simulink model "FInal_Liu_simulation"  (R2023b)
settings: Solver=ode5  StartTime=0.0  StopTime=2  FixedStep=0.0001  RelTol=1e-3
(part 1 of 2)
settings Model: Creator=amaiani  LastModifiedBy=amaiani

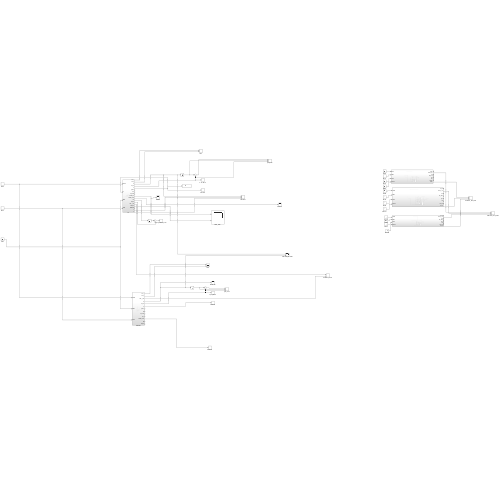
[thumbnail: Simulink's stored preview of the top-level diagram]
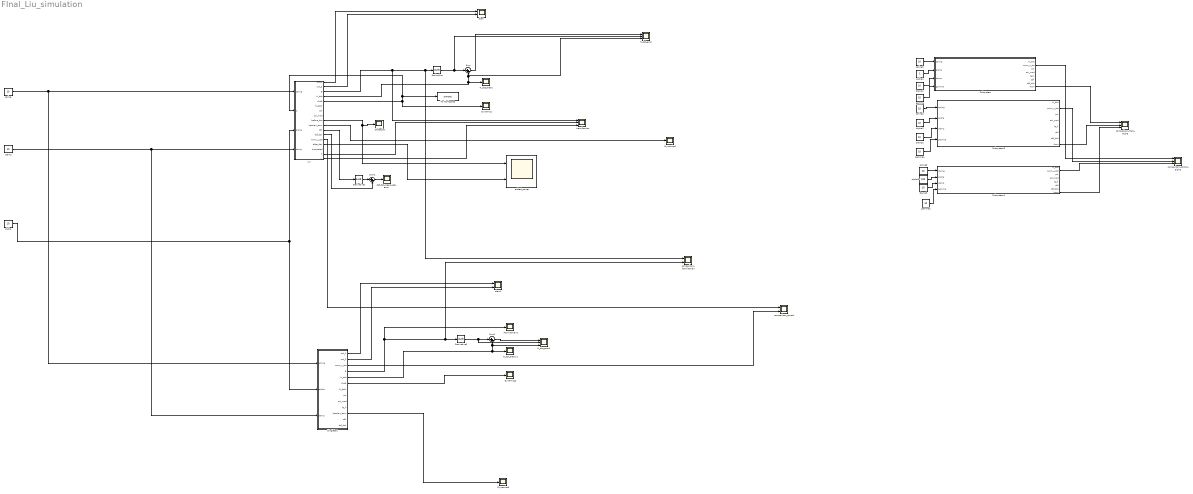
== system FInal_Liu_simulation ==
  Damp{,1..3} (4 alike) : Constant  Value=10
  Derivative : Derivative
  Derivative1 : Derivative
  Derivative2 : Derivative
  Dynamics{,1..3} (4 alike) : Scope
  H_dot_error : Scope  NumInputPorts=3
  H_dot_error1 : Scope  NumInputPorts=3
  H_dot_theory : Scope
  H_dot_theory1 : Scope
  Hamiltonian : Scope  NumInputPorts=3
  Hamiltonian1 : Scope
  Liu : Subsystem
  Singletary : Subsystem
  Subsystem : Subsystem
  Subsystem3 : Subsystem
  Subsystem4 : Subsystem
  Sum : Sum  Inputs=|+-
  Sum1 : Sum  Inputs=|+-
  Sum2 : Sum  Inputs=|+-
  To Workspace : ToWorkspace  VariableName=simout  SampleTime=-1
  added_power : Scope  NumInputPorts=2
  alpha : Constant  Value=10
  alpha1 : Constant
  alpha2 : Constant  Value=10
  alpha3 : Constant  Value=100
  cbf_dot_measured_error : Scope
  comparison_Ham_alpha : Scope  NumInputPorts=3
  comparison_control : Scope  NumInputPorts=2
  comparison_control_alpha : Scope  NumInputPorts=3
  comparison_hamiltonian : Scope  NumInputPorts=2
  dhdqqdot : Scope
  gamma : Constant  Value=10
  gamma1 : Constant  Value=10
  gamma2 : Constant  Value=10
  skew : Scope  NumInputPorts=2
  skew1 : Scope  NumInputPorts=2
  spring{,1..3} (4 alike) : Constant  Value=10
  wires:
  Derivative/1 -> H_dot_error/2, Sum/1
  Sum/1 -> H_dot_error/1
  spring/1 -> Liu/1(spring), Singletary/1(spring)
  Derivative2/1 -> H_dot_error1/2, Sum1/1
  Damp/1 -> Liu/4(damp), Singletary/3(damp)
  Sum1/1 -> H_dot_error1/1
  alpha/1 -> Singletary/2(alpha), Liu/3(alpha)
  Singletary/5(H_dot) -> H_dot_theory1/1, H_dot_error1/3, Sum1/2
  Singletary/4(E) -> Derivative2/1, comparison_hamiltonian/2, Hamiltonian1/1
  Singletary/1(out_1) -> skew1/1
  Singletary/2(out_2) -> skew1/2
  Singletary/3(norm_u_tot) -> comparison_control/2
  Singletary/6(Out6) -> Dynamics2/1
  Singletary/11(hessian_term) -> Dynamics3/1
  Liu/4(H_dot) -> H_dot_theory/1, H_dot_error/3, Sum/2
  Liu/5(Out5) -> Dynamics/1, Liu/2(q), To Workspace/1
  Liu/3(E) -> Derivative/1, comparison_hamiltonian/1, Hamiltonian/1
  Liu/1(out_1) -> skew/1
  Liu/2(out_2) -> skew/2
  Liu/10(hessian_term) -> Dynamics1/1
  Liu/13(norm_u_tot) -> comparison_control/1
  spring1/1 -> Subsystem/1(spring)
  alpha1/1 -> Subsystem/2(alpha)
  Damp1/1 -> Subsystem/3(damp)
  alpha2/1 -> Subsystem3/2(alpha)
  Damp2/1 -> Subsystem3/3(damp)
  spring2/1 -> Subsystem3/1(spring)
  Damp3/1 -> Subsystem4/3(damp)
  alpha3/1 -> Subsystem4/2(alpha)
  spring3/1 -> Subsystem4/1(spring)
  Subsystem/8(Ham) -> comparison_Ham_alpha/1
  Subsystem3/8(Ham) -> comparison_Ham_alpha/2
  Subsystem4/8(Ham) -> comparison_Ham_alpha/3
  Subsystem4/2(norm_u_tot) -> comparison_control_alpha/3
  Subsystem3/2(norm_u_tot) -> comparison_control_alpha/2
  Subsystem/2(norm_u_tot) -> comparison_control_alpha/1
  gamma/1 -> Subsystem/4(gamma)
  gamma1/1 -> Subsystem3/4(gamma)
  gamma2/1 -> Subsystem4/4(gamma)
  Liu/9(before_dot) -> added_power/1, dhdqqdot/1
  Liu/11(cbf) -> Derivative1/1
  Derivative1/1 -> Sum2/1
  Sum2/1 -> cbf_dot_measured_error/1
  Liu/12(cbf_dot) -> Sum2/2
  Liu/14(after_dot) -> added_power/2
  Liu/16(T) -> Hamiltonian/2
  Liu/17(V) -> Hamiltonian/3

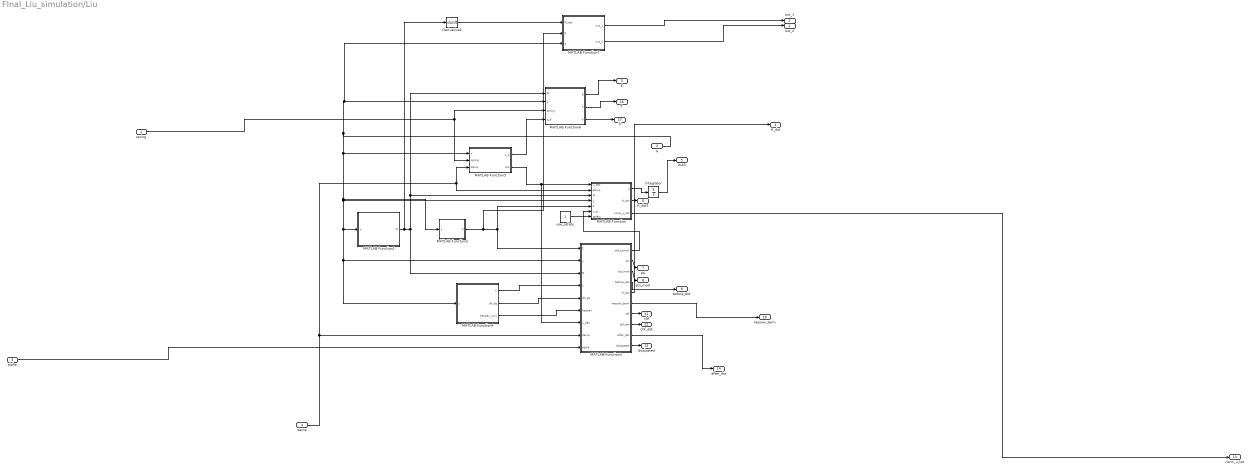
== system FInal_Liu_simulation/Liu ==
  spring : Inport
  q : Inport  Port=2
  alpha : Inport  Port=3
  damp : Inport  Port=4
  Derivative1 : Derivative
  Integrator : Integrator  InitialCondition=[0;0;0;0;0;0]
  MATLAB Function : MATLAB Function  TreatAsAtomicUnit=on
  MATLAB Function1 : MATLAB Function  StartFcn=|  TreatAsAtomicUnit=on
      | % Define numerical values for the parameters
      | xc = 2.5;
      | yc = 2;
      | r = 1;
      | gamma = 2;
      | alpha = 20;
      | 
      | 
      | m1 = 1;
      | m2 = 1;
      | m3 = 1;
      | 
      | 
      | l1 = 1;
      | l2 = 1;
      | l3 = 1;
  MATLAB Function2 : MATLAB Function  StartFcn=|  TreatAsAtomicUnit=on
      | % Define numerical values for the parameters
      | xc = 2.5;
      | yc = 2;
      | r = 1;
      | gamma = 2;
      | alpha = 20;
      | 
      | 
      | m1 = 1;
      | m2 = 1;
      | m3 = 1;
      | 
      | 
      | l1 = 1;
      | l2 = 1;
      | l3 = 1;
  MATLAB Function3 : MATLAB Function  TreatAsAtomicUnit=on
  MATLAB Function4 : MATLAB Function  TreatAsAtomicUnit=on
  MATLAB Function5 : MATLAB Function  TreatAsAtomicUnit=on
  MATLAB Function6 : MATLAB Function  TreatAsAtomicUnit=on
  MATLAB Function7 : MATLAB Function  StartFcn=|  TreatAsAtomicUnit=on
      | % Define numerical values for the parameters
      | xc = 2.5;
      | yc = 2;
      | r = 1;
      | gamma = 2;
      | alpha = 20;
      | 
      | 
      | m1 = 1;
      | m2 = 1;
      | m3 = 1;
      | 
      | 
      | l1 = 1;
      | l2 = 1;
      | l3 = 1;
  use_safety : Constant
  out_1 : Outport
  out_2 : Outport  Port=2
  E : Outport  Port=3
  H_dot : Outport  Port=4
  Out5 : Outport  Port=5
  H_dot1 : Outport  Port=6
  psi : Outport  Port=7
  psi_mod : Outport  Port=8
  before_dot : Outport  Port=9
  hessian_term : Outport  Port=10
  cbf : Outport  Port=11
  cbf_dot : Outport  Port=12
  norm_u_tot : Outport  Port=13
  after_dot : Outport  Port=14
  dissipated : Outport  Port=15
  T : Outport  Port=16
  V : Outport  Port=17
  wires:
  MATLAB Function3/8(cbf_dot) -> cbf_dot/1
  MATLAB Function3/2(psi) -> psi/1
  MATLAB Function3/7(cbf) -> cbf/1
  MATLAB Function/3(norm_u_tot) -> norm_u_tot/1
  MATLAB Function/2(H_dot) -> H_dot1/1
  Integrator/1 -> Out5/1
  MATLAB Function4/3(hessian_sym) -> MATLAB Function3/6(hessian)
  MATLAB Function1/1(M) -> Derivative1/1, MATLAB Function6/1(M), MATLAB Function/3(M), MATLAB Function3/3(M)
  MATLAB Function4/2(dh_dq) -> MATLAB Function3/5(dh_dq)
  MATLAB Function7/1(out_1) -> out_1/1
  alpha/1 -> MATLAB Function3/9(alpha)
  MATLAB Function6/1(E) -> E/1
  MATLAB Function3/3(psi_mod) -> psi_mod/1
  MATLAB Function7/2(out_2) -> out_2/1
  use_safety/1 -> MATLAB Function/7(safety)
  MATLAB Function3/4(before_dot) -> before_dot/1
  Derivative1/1 -> MATLAB Function7/1(M_dot)
  MATLAB Function5/1(q_d) -> MATLAB Function6/4(q_d)
  MATLAB Function3/5(H_dot) -> H_dot/1
  MATLAB Function/1(y) -> Integrator/1
  MATLAB Function3/1(cbf_control) -> MATLAB Function/6(u_sc)
  MATLAB Function2/1(C) -> MATLAB Function/5(C), MATLAB Function3/1(C), MATLAB Function7/2(S)
  MATLAB Function4/1(h) -> MATLAB Function3/4(h)
  spring/1 -> MATLAB Function6/3(spring), MATLAB Function5/2(spring)
  MATLAB Function5/2(out) -> MATLAB Function3/7(u_des), MATLAB Function/1(u_des)
  MATLAB Function3/6(hessian_term) -> hessian_term/1
  q/1 -> MATLAB Function7/3(q), MATLAB Function6/2(y), MATLAB Function5/1(y), MATLAB Function2/1(y), MATLAB Function4/1(y), MATLAB Function3/2(y), MATLAB Function1/1(y), MATLAB Function/4("y ")
  damp/1 -> MATLAB Function/2(damp), MATLAB Function5/3(damp), MATLAB Function3/8(damp)
  MATLAB Function3/9(after_dot) -> after_dot/1
  MATLAB Function3/10(dissipated) -> dissipated/1
  MATLAB Function6/2(T) -> T/1
  MATLAB Function6/3(V) -> V/1

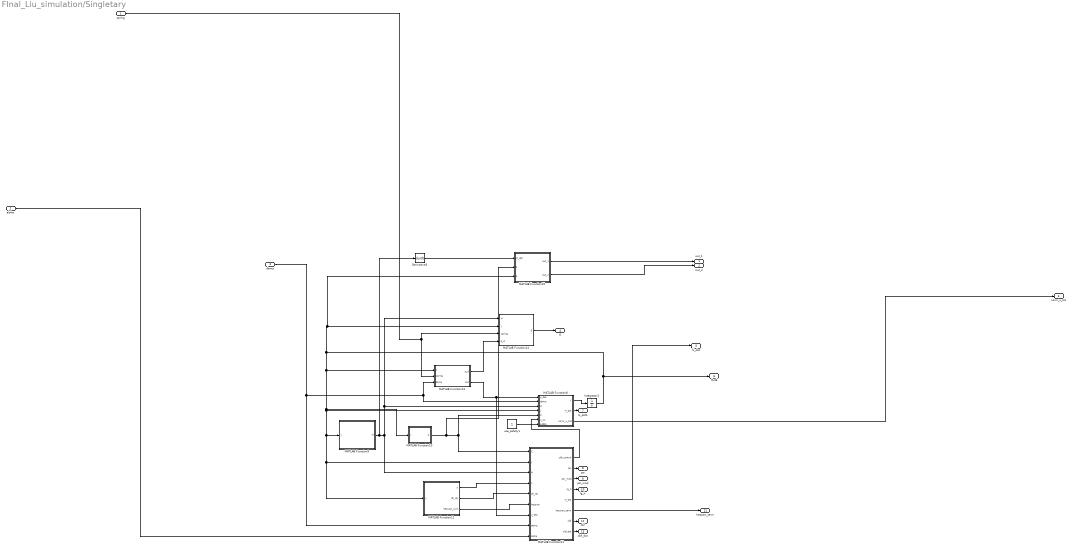
== system FInal_Liu_simulation/Singletary ==
  spring : Inport
  alpha : Inport  Port=2
  damp : Inport  Port=3
  Derivative3 : Derivative
  Integrator1 : Integrator  InitialCondition=[0;0;0;0;0;0]
  MATLAB Function10 : MATLAB Function  StartFcn=|  TreatAsAtomicUnit=on
      | % Define numerical values for the parameters
      | xc = 2.5;
      | yc = 2;
      | r = 1;
      | gamma = 2;
      | alpha = 20;
      | 
      | 
      | m1 = 1;
      | m2 = 1;
      | m3 = 1;
      | 
      | 
      | l1 = 1;
      | l2 = 1;
      | l3 = 1;
  MATLAB Function11 : MATLAB Function  TreatAsAtomicUnit=on
  MATLAB Function12 : MATLAB Function  TreatAsAtomicUnit=on
  MATLAB Function13 : MATLAB Function  TreatAsAtomicUnit=on
  MATLAB Function14 : MATLAB Function  TreatAsAtomicUnit=on
  MATLAB Function15 : MATLAB Function  StartFcn=|  TreatAsAtomicUnit=on
      | % Define numerical values for the parameters
      | xc = 2.5;
      | yc = 2;
      | r = 1;
      | gamma = 2;
      | alpha = 20;
      | 
      | 
      | m1 = 1;
      | m2 = 1;
      | m3 = 1;
      | 
      | 
      | l1 = 1;
      | l2 = 1;
      | l3 = 1;
  MATLAB Function8 : MATLAB Function  TreatAsAtomicUnit=on
  MATLAB Function9 : MATLAB Function  StartFcn=|  TreatAsAtomicUnit=on
      | % Define numerical values for the parameters
      | xc = 2.5;
      | yc = 2;
      | r = 1;
      | gamma = 2;
      | alpha = 20;
      | 
      | 
      | m1 = 1;
      | m2 = 1;
      | m3 = 1;
      | 
      | 
      | l1 = 1;
      | l2 = 1;
      | l3 = 1;
  use_safety1 : Constant
  out_1 : Outport
  out_2 : Outport  Port=2
  norm_u_tot : Outport  Port=3
  E : Outport  Port=4
  H_dot : Outport  Port=5
  Out6 : Outport  Port=6
  H_dot1 : Outport  Port=7
  psi : Outport  Port=8
  psi_mod : Outport  Port=9
  lg_h : Outport  Port=10
  hessian_term : Outport  Port=11
  cbf : Outport  Port=12
  cbf_dot : Outport  Port=13
  wires:
  MATLAB Function11/2(psi) -> psi/1
  MATLAB Function11/4(lg_h) -> lg_h/1
  MATLAB Function11/7(cbf) -> cbf/1
  MATLAB Function8/2(H_dot) -> H_dot1/1
  MATLAB Function11/5(H_dot) -> H_dot/1
  MATLAB Function11/6(hessian_term) -> hessian_term/1
  MATLAB Function14/1(E) -> E/1
  MATLAB Function8/3(norm_u_tot) -> norm_u_tot/1
  MATLAB Function12/3(hessian_sym) -> MATLAB Function11/6(hessian)
  Derivative3/1 -> MATLAB Function15/1(M_dot)
  MATLAB Function12/1(h) -> MATLAB Function11/4(h)
  MATLAB Function8/1(y) -> Integrator1/1
  MATLAB Function11/3(psi_mod) -> psi_mod/1
  alpha/1 -> MATLAB Function11/9(alpha)
  spring/1 -> MATLAB Function13/2(spring), MATLAB Function14/3(spring)
  MATLAB Function10/1(C) -> MATLAB Function8/5(C), MATLAB Function11/1(C), MATLAB Function15/2(S)
  MATLAB Function13/1(q_d) -> MATLAB Function14/4(q_d)
  MATLAB Function11/1(cbf_control) -> MATLAB Function8/6(u_sc)
  MATLAB Function15/2(out_2) -> out_2/1
  Integrator1/1 -> Out6/1, MATLAB Function15/3(q), MATLAB Function14/2(y), MATLAB Function13/1(y), MATLAB Function10/1(y), MATLAB Function12/1(y), MATLAB Function11/2(y), MATLAB Function9/1(y), MATLAB Function8/4("y ")
  MATLAB Function15/1(out_1) -> out_1/1
  damp/1 -> MATLAB Function11/8(damp), MATLAB Function8/2(damp), MATLAB Function13/3(damp)
  MATLAB Function12/2(dh_dq) -> MATLAB Function11/5(dh_dq)
  MATLAB Function13/2(out) -> MATLAB Function11/7(u_des), MATLAB Function8/1(u_des)
  MATLAB Function11/8(cbf_dot) -> cbf_dot/1
  use_safety1/1 -> MATLAB Function8/7(safety)
  MATLAB Function9/1(M) -> Derivative3/1, MATLAB Function14/1(M), MATLAB Function8/3(M), MATLAB Function11/3(M)

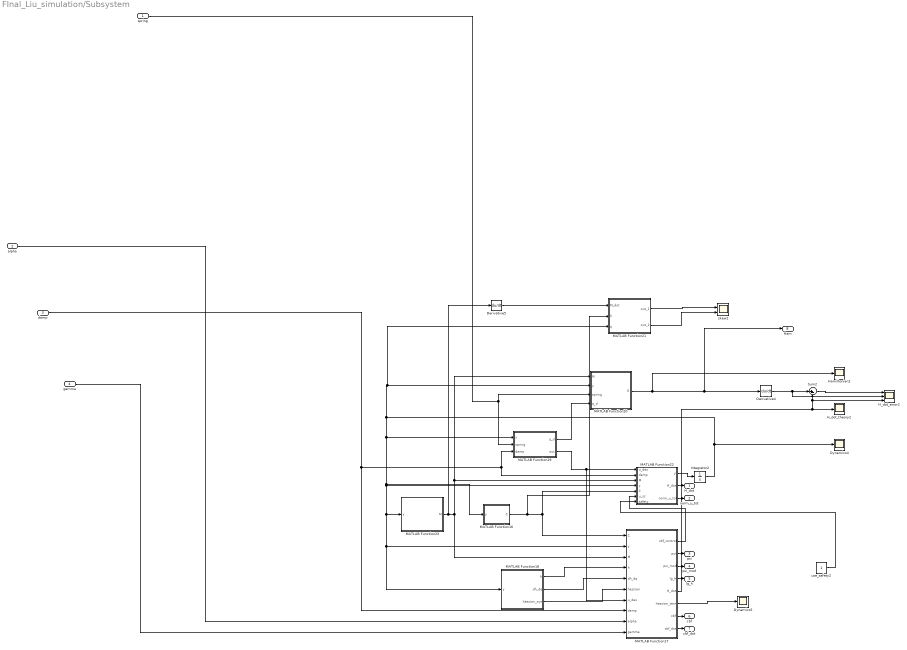
== system FInal_Liu_simulation/Subsystem ==
  spring : Inport
  alpha : Inport  Port=2
  damp : Inport  Port=3
  gamma : Inport  Port=4
  Derivative4 : Derivative
  Derivative5 : Derivative
  Dynamics4 : Scope
  Dynamics5 : Scope
  H_dot_error2 : Scope  NumInputPorts=3
  H_dot_theory2 : Scope
  Hamiltonian2 : Scope
  Integrator2 : Integrator  InitialCondition=[0;0;0;0;0;0]
  MATLAB Function16 : MATLAB Function  StartFcn=|  TreatAsAtomicUnit=on
      | % Define numerical values for the parameters
      | xc = 2.5;
      | yc = 2;
      | r = 1;
      | gamma = 2;
      | alpha = 20;
      | 
      | 
      | m1 = 1;
      | m2 = 1;
      | m3 = 1;
      | 
      | 
      | l1 = 1;
      | l2 = 1;
      | l3 = 1;
  MATLAB Function17 : MATLAB Function  TreatAsAtomicUnit=on
  MATLAB Function18 : MATLAB Function  TreatAsAtomicUnit=on
  MATLAB Function19 : MATLAB Function  TreatAsAtomicUnit=on
  MATLAB Function20 : MATLAB Function  TreatAsAtomicUnit=on
  MATLAB Function21 : MATLAB Function  StartFcn=|  TreatAsAtomicUnit=on
      | % Define numerical values for the parameters
      | xc = 2.5;
      | yc = 2;
      | r = 1;
      | gamma = 2;
      | alpha = 20;
      | 
      | 
      | m1 = 1;
      | m2 = 1;
      | m3 = 1;
      | 
      | 
      | l1 = 1;
      | l2 = 1;
      | l3 = 1;
  MATLAB Function22 : MATLAB Function  TreatAsAtomicUnit=on
  MATLAB Function23 : MATLAB Function  StartFcn=|  TreatAsAtomicUnit=on
      | % Define numerical values for the parameters
      | xc = 2.5;
      | yc = 2;
      | r = 1;
      | gamma = 2;
      | alpha = 20;
      | 
      | 
      | m1 = 1;
      | m2 = 1;
      | m3 = 1;
      | 
      | 
      | l1 = 1;
      | l2 = 1;
      | l3 = 1;
  Sum2 : Sum  Inputs=|+-
  skew2 : Scope  NumInputPorts=2
  use_safety2 : Constant
  H_dot : Outport
  norm_u_tot : Outport  Port=2
  psi : Outport  Port=3
  psi_mod : Outport  Port=4
  lg_h : Outport  Port=5
  cbf : Outport  Port=6
  cbf_dot : Outport  Port=7
  Ham : Outport  Port=8
  wires:
  MATLAB Function17/3(psi_mod) -> psi_mod/1
  MATLAB Function17/8(cbf_dot) -> cbf_dot/1
  MATLAB Function17/4(lg_h) -> lg_h/1
  alpha/1 -> MATLAB Function17/9(alpha)
  MATLAB Function17/2(psi) -> psi/1
  MATLAB Function17/1(cbf_control) -> MATLAB Function22/6(u_sc)
  MATLAB Function23/1(M) -> Derivative5/1, MATLAB Function20/1(M), MATLAB Function22/3(M), MATLAB Function17/3(M)
  use_safety2/1 -> MATLAB Function22/7(safety)
  MATLAB Function22/1(y) -> Integrator2/1
  MATLAB Function17/7(cbf) -> cbf/1
  Sum2/1 -> H_dot_error2/1
  Derivative4/1 -> H_dot_error2/2, Sum2/1
  MATLAB Function22/3(norm_u_tot) -> norm_u_tot/1
  MATLAB Function18/2(dh_dq) -> MATLAB Function17/5(dh_dq)
  Derivative5/1 -> MATLAB Function21/1(M_dot)
  MATLAB Function19/2(out) -> MATLAB Function17/7(u_des), MATLAB Function22/1(u_des)
  MATLAB Function17/6(hessian_term) -> Dynamics5/1
  MATLAB Function18/3(hessian_sym) -> MATLAB Function17/6(hessian)
  MATLAB Function21/1(out_1) -> skew2/1
  MATLAB Function21/2(out_2) -> skew2/2
  MATLAB Function19/1(q_d) -> MATLAB Function20/4(q_d)
  MATLAB Function22/2(H_dot) -> H_dot/1
  damp/1 -> MATLAB Function17/8(damp), MATLAB Function22/2(damp), MATLAB Function19/3(damp)
  MATLAB Function20/1(E) -> Ham/1, Derivative4/1, Hamiltonian2/1
  Integrator2/1 -> Dynamics4/1, MATLAB Function21/3(q), MATLAB Function20/2(y), MATLAB Function19/1(y), MATLAB Function16/1(y), MATLAB Function18/1(y), MATLAB Function17/2(y), MATLAB Function23/1(y), MATLAB Function22/4("y ")
  MATLAB Function18/1(h) -> MATLAB Function17/4(h)
  spring/1 -> MATLAB Function19/2(spring), MATLAB Function20/3(spring)
  MATLAB Function16/1(C) -> MATLAB Function22/5(C), MATLAB Function17/1(C), MATLAB Function21/2(S)
  MATLAB Function17/5(H_dot) -> H_dot_theory2/1, H_dot_error2/3, Sum2/2
  gamma/1 -> MATLAB Function17/10(gamma)

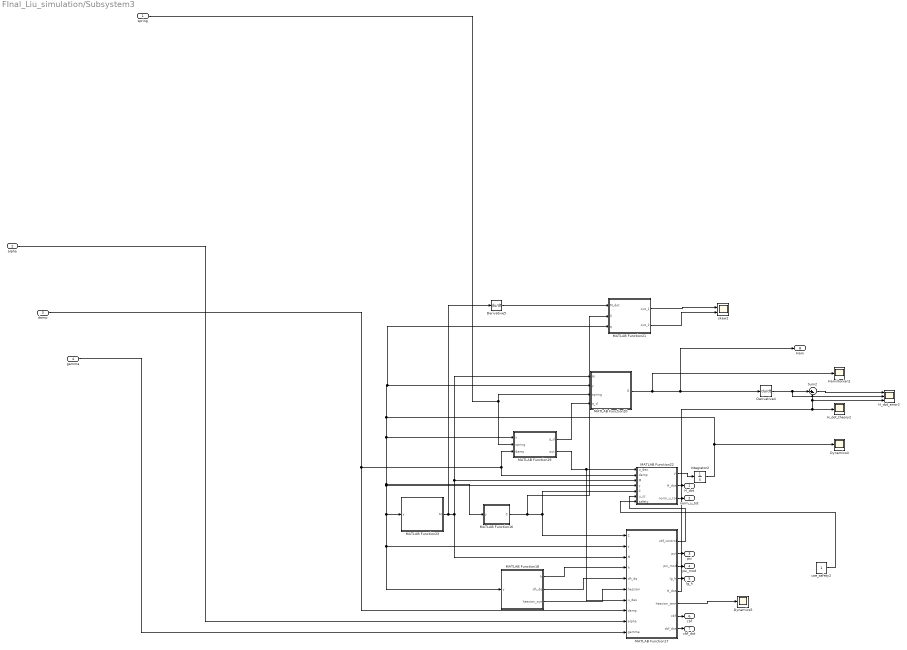
== system FInal_Liu_simulation/Subsystem3 ==
  spring : Inport
  alpha : Inport  Port=2
  damp : Inport  Port=3
  gamma : Inport  Port=4
  Derivative4 : Derivative
  Derivative5 : Derivative
  Dynamics4 : Scope
  Dynamics5 : Scope
  H_dot_error2 : Scope  NumInputPorts=3
  H_dot_theory2 : Scope
  Hamiltonian2 : Scope
  Integrator2 : Integrator  InitialCondition=[0;0;0;0;0;0]
  MATLAB Function16 : MATLAB Function  StartFcn=|  TreatAsAtomicUnit=on
      | % Define numerical values for the parameters
      | xc = 2.5;
      | yc = 2;
      | r = 1;
      | gamma = 2;
      | alpha = 20;
      | 
      | 
      | m1 = 1;
      | m2 = 1;
      | m3 = 1;
      | 
      | 
      | l1 = 1;
      | l2 = 1;
      | l3 = 1;
  MATLAB Function17 : MATLAB Function  TreatAsAtomicUnit=on
  MATLAB Function18 : MATLAB Function  TreatAsAtomicUnit=on
  MATLAB Function19 : MATLAB Function  TreatAsAtomicUnit=on
  MATLAB Function20 : MATLAB Function  TreatAsAtomicUnit=on
  MATLAB Function21 : MATLAB Function  StartFcn=|  TreatAsAtomicUnit=on
      | % Define numerical values for the parameters
      | xc = 2.5;
      | yc = 2;
      | r = 1;
      | gamma = 2;
      | alpha = 20;
      | 
      | 
      | m1 = 1;
      | m2 = 1;
      | m3 = 1;
      | 
      | 
      | l1 = 1;
      | l2 = 1;
      | l3 = 1;
  MATLAB Function22 : MATLAB Function  TreatAsAtomicUnit=on
  MATLAB Function23 : MATLAB Function  StartFcn=|  TreatAsAtomicUnit=on
      | % Define numerical values for the parameters
      | xc = 2.5;
      | yc = 2;
      | r = 1;
      | gamma = 2;
      | alpha = 20;
      | 
      | 
      | m1 = 1;
      | m2 = 1;
      | m3 = 1;
      | 
      | 
      | l1 = 1;
      | l2 = 1;
      | l3 = 1;
  Sum2 : Sum  Inputs=|+-
  skew2 : Scope  NumInputPorts=2
  use_safety2 : Constant
  H_dot : Outport
  norm_u_tot : Outport  Port=2
  psi : Outport  Port=3
  psi_mod : Outport  Port=4
  lg_h : Outport  Port=5
  cbf : Outport  Port=6
  cbf_dot : Outport  Port=7
  Ham : Outport  Port=8
  wires:
  MATLAB Function17/3(psi_mod) -> psi_mod/1
  MATLAB Function17/8(cbf_dot) -> cbf_dot/1
  MATLAB Function17/4(lg_h) -> lg_h/1
  alpha/1 -> MATLAB Function17/9(alpha)
  MATLAB Function17/2(psi) -> psi/1
  MATLAB Function17/1(cbf_control) -> MATLAB Function22/6(u_sc)
  MATLAB Function23/1(M) -> Derivative5/1, MATLAB Function20/1(M), MATLAB Function22/3(M), MATLAB Function17/3(M)
  use_safety2/1 -> MATLAB Function22/7(safety)
  MATLAB Function22/1(y) -> Integrator2/1
  MATLAB Function17/7(cbf) -> cbf/1
  Sum2/1 -> H_dot_error2/1
  Derivative4/1 -> H_dot_error2/2, Sum2/1
  MATLAB Function22/3(norm_u_tot) -> norm_u_tot/1
  MATLAB Function18/2(dh_dq) -> MATLAB Function17/5(dh_dq)
  Derivative5/1 -> MATLAB Function21/1(M_dot)
  MATLAB Function19/2(out) -> MATLAB Function17/7(u_des), MATLAB Function22/1(u_des)
  MATLAB Function17/6(hessian_term) -> Dynamics5/1
  MATLAB Function18/3(hessian_sym) -> MATLAB Function17/6(hessian)
  MATLAB Function21/1(out_1) -> skew2/1
  MATLAB Function21/2(out_2) -> skew2/2
  MATLAB Function19/1(q_d) -> MATLAB Function20/4(q_d)
  MATLAB Function22/2(H_dot) -> H_dot/1
  damp/1 -> MATLAB Function17/8(damp), MATLAB Function22/2(damp), MATLAB Function19/3(damp)
  MATLAB Function20/1(E) -> Ham/1, Derivative4/1, Hamiltonian2/1
  Integrator2/1 -> Dynamics4/1, MATLAB Function21/3(q), MATLAB Function20/2(y), MATLAB Function19/1(y), MATLAB Function16/1(y), MATLAB Function18/1(y), MATLAB Function17/2(y), MATLAB Function23/1(y), MATLAB Function22/4("y ")
  MATLAB Function18/1(h) -> MATLAB Function17/4(h)
  spring/1 -> MATLAB Function19/2(spring), MATLAB Function20/3(spring)
  MATLAB Function16/1(C) -> MATLAB Function22/5(C), MATLAB Function17/1(C), MATLAB Function21/2(S)
  MATLAB Function17/5(H_dot) -> H_dot_theory2/1, H_dot_error2/3, Sum2/2
  gamma/1 -> MATLAB Function17/10(gamma)

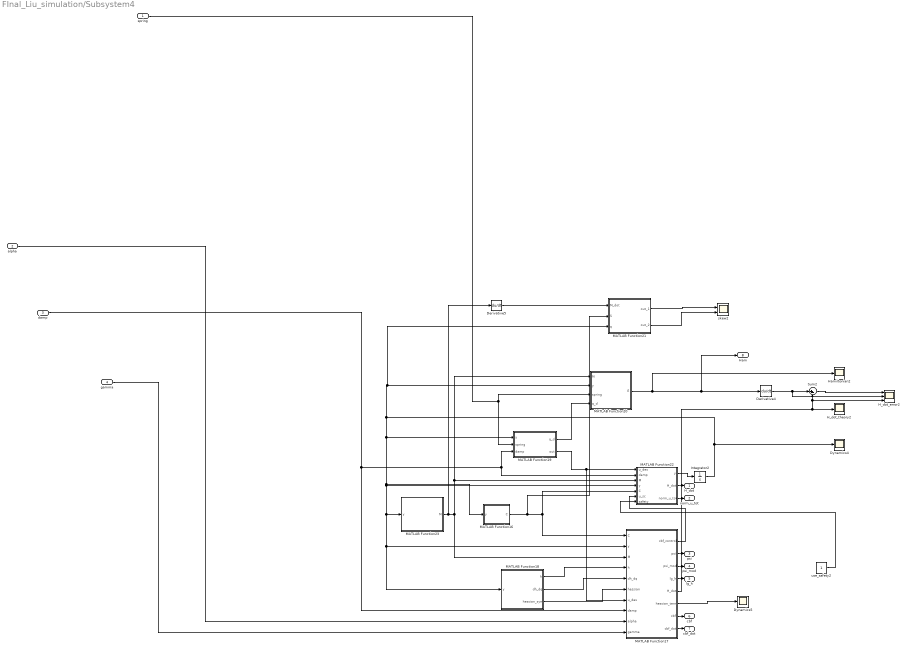
== system FInal_Liu_simulation/Subsystem4 ==
  spring : Inport
  alpha : Inport  Port=2
  damp : Inport  Port=3
  gamma : Inport  Port=4
  Derivative4 : Derivative
  Derivative5 : Derivative
  Dynamics4 : Scope
  Dynamics5 : Scope
  H_dot_error2 : Scope  NumInputPorts=3
  H_dot_theory2 : Scope
  Hamiltonian2 : Scope
  Integrator2 : Integrator  InitialCondition=[0;0;0;0;0;0]
  MATLAB Function16 : MATLAB Function  StartFcn=|  TreatAsAtomicUnit=on
      | % Define numerical values for the parameters
      | xc = 2.5;
      | yc = 2;
      | r = 1;
      | gamma = 2;
      | alpha = 20;
      | 
      | 
      | m1 = 1;
      | m2 = 1;
      | m3 = 1;
      | 
      | 
      | l1 = 1;
      | l2 = 1;
      | l3 = 1;
  MATLAB Function17 : MATLAB Function  TreatAsAtomicUnit=on
  MATLAB Function18 : MATLAB Function  TreatAsAtomicUnit=on
  MATLAB Function19 : MATLAB Function  TreatAsAtomicUnit=on
  MATLAB Function20 : MATLAB Function  TreatAsAtomicUnit=on
  MATLAB Function21 : MATLAB Function  StartFcn=|  TreatAsAtomicUnit=on
      | % Define numerical values for the parameters
      | xc = 2.5;
      | yc = 2;
      | r = 1;
      | gamma = 2;
      | alpha = 20;
      | 
      | 
      | m1 = 1;
      | m2 = 1;
      | m3 = 1;
      | 
      | 
      | l1 = 1;
      | l2 = 1;
      | l3 = 1;
  MATLAB Function22 : MATLAB Function  TreatAsAtomicUnit=on
  MATLAB Function23 : MATLAB Function  StartFcn=|  TreatAsAtomicUnit=on
      | % Define numerical values for the parameters
      | xc = 2.5;
      | yc = 2;
      | r = 1;
      | gamma = 2;
      | alpha = 20;
      | 
      | 
      | m1 = 1;
      | m2 = 1;
      | m3 = 1;
      | 
      | 
      | l1 = 1;
      | l2 = 1;
      | l3 = 1;
  Sum2 : Sum  Inputs=|+-
  skew2 : Scope  NumInputPorts=2
  use_safety2 : Constant
  H_dot : Outport
  norm_u_tot : Outport  Port=2
  psi : Outport  Port=3
  psi_mod : Outport  Port=4
  lg_h : Outport  Port=5
  cbf : Outport  Port=6
  cbf_dot : Outport  Port=7
  Ham : Outport  Port=8
  wires:
  MATLAB Function17/3(psi_mod) -> psi_mod/1
  MATLAB Function17/8(cbf_dot) -> cbf_dot/1
  MATLAB Function17/4(lg_h) -> lg_h/1
  alpha/1 -> MATLAB Function17/9(alpha)
  MATLAB Function17/2(psi) -> psi/1
  MATLAB Function17/1(cbf_control) -> MATLAB Function22/6(u_sc)
  MATLAB Function23/1(M) -> Derivative5/1, MATLAB Function20/1(M), MATLAB Function22/3(M), MATLAB Function17/3(M)
  use_safety2/1 -> MATLAB Function22/7(safety)
  MATLAB Function22/1(y) -> Integrator2/1
  MATLAB Function17/7(cbf) -> cbf/1
  Sum2/1 -> H_dot_error2/1
  Derivative4/1 -> H_dot_error2/2, Sum2/1
  MATLAB Function22/3(norm_u_tot) -> norm_u_tot/1
  MATLAB Function18/2(dh_dq) -> MATLAB Function17/5(dh_dq)
  Derivative5/1 -> MATLAB Function21/1(M_dot)
  MATLAB Function19/2(out) -> MATLAB Function17/7(u_des), MATLAB Function22/1(u_des)
  MATLAB Function17/6(hessian_term) -> Dynamics5/1
  MATLAB Function18/3(hessian_sym) -> MATLAB Function17/6(hessian)
  MATLAB Function21/1(out_1) -> skew2/1
  MATLAB Function21/2(out_2) -> skew2/2
  MATLAB Function19/1(q_d) -> MATLAB Function20/4(q_d)
  MATLAB Function22/2(H_dot) -> H_dot/1
  damp/1 -> MATLAB Function17/8(damp), MATLAB Function22/2(damp), MATLAB Function19/3(damp)
  MATLAB Function20/1(E) -> Ham/1, Derivative4/1, Hamiltonian2/1
  Integrator2/1 -> Dynamics4/1, MATLAB Function21/3(q), MATLAB Function20/2(y), MATLAB Function19/1(y), MATLAB Function16/1(y), MATLAB Function18/1(y), MATLAB Function17/2(y), MATLAB Function23/1(y), MATLAB Function22/4("y ")
  MATLAB Function18/1(h) -> MATLAB Function17/4(h)
  spring/1 -> MATLAB Function19/2(spring), MATLAB Function20/3(spring)
  MATLAB Function16/1(C) -> MATLAB Function22/5(C), MATLAB Function17/1(C), MATLAB Function21/2(S)
  MATLAB Function17/5(H_dot) -> H_dot_theory2/1, H_dot_error2/3, Sum2/2
  gamma/1 -> MATLAB Function17/10(gamma)

== matlab function FInal_Liu_simulation/Liu/MATLAB Function6 ==
  data: M input; E output; y input; spring input; q_d input; T output; V output
function [E,T,V] = energy(M,y,spring, q_d)
    q = y(1:3);
    dq = y(4:6);
    
    T = 0.5 * (dq' * M * dq) ;
    V =0.5 * spring *(q-q_d)' * (q-q_d);
    E = T + V;

== matlab function FInal_Liu_simulation/Liu/MATLAB Function7 ==
  data: M_dot input; out_1 output; S input; q input; out_2 output


function [out_1, out_2] = M_dot_coriolis_check(M_dot,S, q)
    dq = reshape(q(4:6),[3,1]);
    
    q1 = q(1);
    q2 = q(2);
    q3 = q(3);
    dq1 = q(4);
    dq2 = q(5);
    dq3 = q(6);

    check = M_dot - 2 * S;


    out_1 = dq' * check * dq;


    M_dot_formula =   [        - dq2*(sin(q2 + q3) + 3*sin(q2)) - dq3*(sin(q2 + q3) + sin(q3)), - dq3*(sin(q2 + q3)/2 + sin(q3)) - dq2*(sin(q2 + q3)/2 + (3*sin(q2))/2), - (dq2*sin(q2 + q3))/2 - dq3*(sin(q2 + q3)/2 + sin(q3)/2);
- dq3*(sin(q2 + q3)/2 + sin(q3)) - dq2*(sin(q2 + q3)/2 + (3*sin(q2))/2),                                                            -dq3*sin(q3),                                          -(dq3*sin(q3))/2;
              - (dq2*sin(q2 + q3))/2 - dq3*(sin(q2 + q3)/2 + sin(q3)/2),                                                        -(dq3*sin(q3))/2,                                                         0];
 

    
    out_2 = dq' * (M_dot_formula - 2 * S) * dq;
end

== matlab function FInal_Liu_simulation/Singletary/MATLAB Function10 ==
  data: y input; C output
function C = coriolis(y)

    q1 = y(1);
    q2 = y(2);
    q3 = y(3);
    dq1 = y(4);
    dq2 = y(5);
    dq3 = y(6);


    C = [- dq2*(sin(q2 + q3)/2 + (3*sin(q2))/2) - dq3*(sin(q2 + q3)/2 + sin(q3)/2), - dq1*(sin(q2 + q3)/2 + (3*sin(q2))/2) - dq2*(sin(q2 + q3)/2 + (3*sin(q2))/2) - dq3*(sin(q2 + q3)/2 + sin(q3)/2), - dq1*(sin(q2 + q3)/2 + sin(q3)/2) - dq2*(sin(q2 + q3)/2 + sin(q3)/2) - dq3*(sin(q2 + q3)/2 + sin(q3)/2);
                dq1*(sin(q2 + q3)/2 + (3*sin(q2))/2) - (dq3*sin(q3))/2,                                                                                                 -(dq3*sin(q3))/2,                                                    - (dq1*sin(q3))/2 - (dq2*sin(q3))/2 - (dq3*sin(q3))/2;
                       dq1*(sin(q2 + q3)/2 + sin(q3)/2) + (dq2*sin(q3))/2,                                                                                (dq1*sin(q3))/2 + (dq2*sin(q3))/2,                                                                                                        0];

== matlab function FInal_Liu_simulation/Singletary/MATLAB Function11 ==
  data: C input; y input; cbf_control output; M input; h input; dh_dq input; hessian input; u_des input; psi output; psi_mod output; lg_h output; H_dot output; damp input; hessian_term output; cbf output; cbf_dot output; alpha input

function [cbf_control, psi, psi_mod,lg_h, H_dot, hessian_term, cbf, cbf_dot]= CBF(C, y, M, h, dh_dq, hessian, u_des, damp, alpha)
% Define numerical values for the parameters
    xc = 2.5;
    yc = 2;
    r = 1;
    gamma = 2;

    
    m1 = 1;
    m2 = 1;
    m3 = 1;
    
    l1 = 1;
    l2 = 1;
    l3 = 1;
    
    q = reshape(y(1:3),[3,1]);
    dq = reshape(y(4:6),[3,1]);
    dh_dq = reshape(dh_dq,[1,3]);

    LIU = 0;

    if LIU == 1

    
        cbf = alpha * h + dh_dq * dq;
        lg_h = zeros(1,3);
        cbf_dot_prior = alpha .* dh_dq * dq + dq' * hessian * dq + dh_dq * (inv(M)* (-C * dq + u_des));
        psi = cbf_dot_prior + gamma .* cbf;
        if psi<0
            lg_h = dh_dq * inv(M);
            cbf_control =  - lg_h' /(lg_h * lg_h')  .* psi;
            
        else
            cbf_control = zeros(3,1);
        end
        cbf_dot = alpha .* dh_dq * dq + dq' * hessian * dq + dh_dq * inv(M)* (-C * dq + u_des+ cbf_control);
        psi_mod = cbf_dot + gamma .* cbf;

        H_dot = dq' * cbf_control - dq' * damp * dq;

        hessian_term = dq' * hessian * dq;
    
    else
        KE = 0.5 * dq' * M * dq;
        cbf = alpha * h - KE;
        lg_h = zeros(1,3);
        cbf_dot_prior = alpha .* dh_dq * dq - dq' * inv(M) * u_des;
        psi = cbf_dot_prior + gamma .* cbf;
        if psi<0
            lg_h = -dq';
            cbf_control =  dq /(dq'*dq)  .* psi;
        else
            cbf_control = zeros(3,1);
        end
        cbf_dot =  alpha .* dh_dq * dq - dq' * inv(M) * (u_des+cbf_control) ;
        psi_mod = cbf_dot + gamma .* cbf;

        H_dot = dq' * cbf_control - dq' * damp * dq;


        hessian_term = 0;
        
    end
    
end

== matlab function FInal_Liu_simulation/Singletary/MATLAB Function12 ==
  data: y input; h output; dh_dq output; hessian_sym output
function [h, dh_dq, hessian_sym] = obstacle(y)
    % Define numerical values for the parameters
    xc = 2.5;
    yc = 2;
    r = 1;

    l1 = 1;
    l2 = 1;
    l3 = 1;
    
    % Compute the end-effector position using forward kinematics
    q1 = y(1);
    q2 = y(2);
    q3 = y(3);
    
    x_ee = l1 * cos(q1) + l2 * cos(q1 + q2) + l3 * cos(q1 + q2 + q3);
    y_ee = l1 * sin(q1) + l2 * sin(q1 + q2) + l3 * sin(q1 + q2 + q3);
    
    % Compute the control barrier function h
    h = (xc - x_ee)^2 + (yc - y_ee)^2 - r^2;
    
    % Define the expressions for dh_dq and hessian_sym
    dh_dq = [2*(cos(q1 + q2 + q3) + cos(q1 + q2) + cos(q1))*(sin(q1 + q2 + q3) + sin(q1 + q2) + sin(q1) - 2) - 2*(sin(q1 + q2 + q3) + sin(q1 + q2) + sin(q1))*(cos(q1 + q2 + q3) + cos(q1 + q2) + cos(q1) - 5/2), 2*(cos(q1 + q2 + q3) + cos(q1 + q2))*(sin(q1 + q2 + q3) + sin(q1 + q2) + sin(q1) - 2) - 2*(sin(q1 + q2 + q3) + sin(q1 + q2))*(cos(q1 + q2 + q3) + cos(q1 + q2) + cos(q1) - 5/2), 2*cos(q1 + q2 + q3)*(sin(q1 + q2 + q3) + sin(q1 + q2) + sin(q1) - 2) - 2*sin(q1 + q2 + q3)*(cos(q1 + q2 + q3) + cos(q1 + q2) + cos(q1) - 5/2)];


    hessian_sym = [                                              2*(cos(q1 + q2 + q3) + cos(q1 + q2) + cos(q1))^2 - 2*(cos(q1 + q2 + q3) + cos(q1 + q2) + cos(q1))*(cos(q1 + q2 + q3) + cos(q1 + q2) + cos(q1) - 5/2) + 2*(sin(q1 + q2 + q3) + sin(q1 + q2) + sin(q1))^2 - 2*(sin(q1 + q2 + q3) + sin(q1 + q2) + sin(q1))*(sin(q1 + q2 + q3) + sin(q1 + q2) + sin(q1) - 2), 2*(cos(q1 + q2 + q3) + cos(q1 + q2))*(cos(q1 + q2 + q3) + cos(q1 + q2) + cos(q1)) - 2*(cos(q1 + q2 + q3) + cos(q1 + q2))*(cos(q1 + q2 + q3) + cos(q1 + q2) + cos(q1) - 5/2) + 2*(sin(q1 + q2 + q3) + sin(q1 + q2))*(sin(q1 + q2 + q3) + sin(q1 + q2) + sin(q1)) - 2*(sin(q1 + q2 + q3) + sin(q1 + q2))*(sin(q1 + q2 + q3) + sin(q1 + q2) + sin(q1) - 2), 2*cos(q1 + q2 + q3)*(cos(q1 + q2 + q3) + cos(q1 + q2) + cos(q1)) - 2*cos(q1 + q2 + q3)*(cos(q1 + q2 + q3) + cos(q1 + q2) + cos(q1) - 5/2) + 2*sin(q1 + q2 + q3)*(sin(q1 + q2 + q3) + sin(q1 + q2) + sin(q1)) - 2*sin(q1 + q2 + q3)*(sin(q1 + q2 + q3) + sin(q1 + q2) + sin(q1) - 2);
        2*(cos(q1 + q2 + q3) + cos(q1 + q2))*(cos(q1 + q2 + q3) + cos(q1 + q2) + cos(q1)) - 2*(cos(q1 + q2 + q3) + cos(q1 + q2))*(cos(q1 + q2 + q3) + cos(q1 + q2) + cos(q1) - 5/2) + 2*(sin(q1 + q2 + q3) + sin(q1 + q2))*(sin(q1 + q2 + q3) + sin(q1 + q2) + sin(q1)) - 2*(sin(q1 + q2 + q3) + sin(q1 + q2))*(sin(q1 + q2 + q3) + sin(q1 + q2) + sin(q1) - 2),                                                                                       2*(cos(q1 + q2 + q3) + cos(q1 + q2))^2 - 2*(cos(q1 + q2 + q3) + cos(q1 + q2))*(cos(q1 + q2 + q3) + cos(q1 + q2) + cos(q1) - 5/2) + 2*(sin(q1 + q2 + q3) + sin(q1 + q2))^2 - 2*(sin(q1 + q2 + q3) + sin(q1 + q2))*(sin(q1 + q2 + q3) + sin(q1 + q2) + sin(q1) - 2),                     2*cos(q1 + q2 + q3)*(cos(q1 + q2 + q3) + cos(q1 + q2)) - 2*cos(q1 + q2 + q3)*(cos(q1 + q2 + q3) + cos(q1 + q2) + cos(q1) - 5/2) - 2*sin(q1 + q2 + q3)*(sin(q1 + q2 + q3) + sin(q1 + q2) + sin(q1) - 2) + 2*sin(q1 + q2 + q3)*(sin(q1 + q2 + q3) + sin(q1 + q2));
                                                                            2*cos(q1 + q2 + q3)*(cos(q1 + q2 + q3) + cos(q1 + q2) + cos(q1)) - 2*cos(q1 + q2 + q3)*(cos(q1 + q2 + q3) + cos(q1 + q2) + cos(q1) - 5/2) + 2*sin(q1 + q2 + q3)*(sin(q1 + q2 + q3) + sin(q1 + q2) + sin(q1)) - 2*sin(q1 + q2 + q3)*(sin(q1 + q2 + q3) + sin(q1 + q2) + sin(q1) - 2),                                                                                         2*cos(q1 + q2 + q3)*(cos(q1 + q2 + q3) + cos(q1 + q2)) - 2*cos(q1 + q2 + q3)*(cos(q1 + q2 + q3) + cos(q1 + q2) + cos(q1) - 5/2) - 2*sin(q1 + q2 + q3)*(sin(q1 + q2 + q3) + sin(q1 + q2) + sin(q1) - 2) + 2*sin(q1 + q2 + q3)*(sin(q1 + q2 + q3) + sin(q1 + q2)),                                                                                       2*cos(q1 + q2 + q3)^2 - 2*cos(q1 + q2 + q3)*(cos(q1 + q2 + q3) + cos(q1 + q2) + cos(q1) - 5/2) + 2*sin(q1 + q2 + q3)^2 - 2*sin(q1 + q2 + q3)*(sin(q1 + q2 + q3) + sin(q1 + q2) + sin(q1) - 2)];
     

    % d = eig(hessian_sym)
    % isposdef = all(d >= 0);
    % 
    % assert(isposdef, 'error hessian');
end

== matlab function FInal_Liu_simulation/Singletary/MATLAB Function13 ==
  data: q_d output; y input; spring input; out output; damp input
function [q_d, out] = u_des(y, spring, damp)


    q = reshape(y(1:3),[3,1]);
    dq = reshape(y(4:6),[3,1]);

    q_d = [pi; 0; pi/4];
    
    out =  - damp * dq - spring * (q-q_d);

== matlab function FInal_Liu_simulation/Singletary/MATLAB Function14 ==
  data: M input; E output; y input; spring input; q_d input
function E = energy(M,y,spring, q_d)
    q = y(1:3);
    dq = y(4:6);
    

    E = 0.5 * (dq' * M * dq) + 0.5 * spring *(q-q_d)' * (q-q_d);

== matlab function FInal_Liu_simulation/Singletary/MATLAB Function15 ==
  data: M_dot input; out_1 output; S input; q input; out_2 output


function [out_1, out_2] = M_dot_coriolis_check(M_dot,S, q)
    dq = reshape(q(4:6),[3,1]);
    
    q1 = q(1);
    q2 = q(2);
    q3 = q(3);
    dq1 = q(4);
    dq2 = q(5);
    dq3 = q(6);

    check = M_dot - 2 * S;


    out_1 = dq' * check * dq;


    M_dot_formula =   [        - dq2*(sin(q2 + q3) + 3*sin(q2)) - dq3*(sin(q2 + q3) + sin(q3)), - dq3*(sin(q2 + q3)/2 + sin(q3)) - dq2*(sin(q2 + q3)/2 + (3*sin(q2))/2), - (dq2*sin(q2 + q3))/2 - dq3*(sin(q2 + q3)/2 + sin(q3)/2);
- dq3*(sin(q2 + q3)/2 + sin(q3)) - dq2*(sin(q2 + q3)/2 + (3*sin(q2))/2),                                                            -dq3*sin(q3),                                          -(dq3*sin(q3))/2;
              - (dq2*sin(q2 + q3))/2 - dq3*(sin(q2 + q3)/2 + sin(q3)/2),                                                        -(dq3*sin(q3))/2,                                                         0];
 

    
    out_2 = dq' * (M_dot_formula - 2 * S) * dq;
end

== matlab function FInal_Liu_simulation/Singletary/MATLAB Function8 ==
  data: u_des input; damp input; M input; y input; y output; C input; H_dot output; u_sc input; safety input; norm_u_tot output
function [y,H_dot,norm_u_tot]= dynamics(u_des, damp , M,y, C, u_sc, safety)
    
    q = reshape(y(1:3),[3,1]);
    dq = reshape(y(4:6),[3,1]);



    [~, p] = chol(M);
    decision = (p == 0);

    assert(decision, 'Inertia matrix is not positive definite');
    
    u_tot = u_des + safety * u_sc;
    norm_u_tot=norm(u_tot);
    ddq = inv(M) * (u_tot - C * dq ); % + u_sc

    H_dot = - dq' * damp * dq;

    y = [dq; ddq];

== matlab function FInal_Liu_simulation/Singletary/MATLAB Function9 ==
  data: y input; M output
function M = inertia_M(y)

    q1 = y(1);
    q2 = y(2);
    q3 = y(3);

    M  = [        cos(q2 + q3) + 3*cos(q2) + cos(q3) + 4, cos(q2 + q3)/2 + (3*cos(q2))/2 + cos(q3) + 5/3, cos(q2 + q3)/2 + cos(q3)/2 + 1/3;
cos(q2 + q3)/2 + (3*cos(q2))/2 + cos(q3) + 5/3,                                  cos(q3) + 5/3,                  cos(q3)/2 + 1/3;
              cos(q2 + q3)/2 + cos(q3)/2 + 1/3,                                cos(q3)/2 + 1/3,                              1/3];

== matlab function FInal_Liu_simulation/Subsystem/MATLAB Function16 ==
  data: y input; C output
function C = coriolis(y)

    q1 = y(1);
    q2 = y(2);
    q3 = y(3);
    dq1 = y(4);
    dq2 = y(5);
    dq3 = y(6);


    C = [- dq2*(sin(q2 + q3)/2 + (3*sin(q2))/2) - dq3*(sin(q2 + q3)/2 + sin(q3)/2), - dq1*(sin(q2 + q3)/2 + (3*sin(q2))/2) - dq2*(sin(q2 + q3)/2 + (3*sin(q2))/2) - dq3*(sin(q2 + q3)/2 + sin(q3)/2), - dq1*(sin(q2 + q3)/2 + sin(q3)/2) - dq2*(sin(q2 + q3)/2 + sin(q3)/2) - dq3*(sin(q2 + q3)/2 + sin(q3)/2);
                dq1*(sin(q2 + q3)/2 + (3*sin(q2))/2) - (dq3*sin(q3))/2,                                                                                                 -(dq3*sin(q3))/2,                                                    - (dq1*sin(q3))/2 - (dq2*sin(q3))/2 - (dq3*sin(q3))/2;
                       dq1*(sin(q2 + q3)/2 + sin(q3)/2) + (dq2*sin(q3))/2,                                                                                (dq1*sin(q3))/2 + (dq2*sin(q3))/2,                                                                                                        0];

== matlab function FInal_Liu_simulation/Subsystem/MATLAB Function17 ==
  data: C input; y input; cbf_control output; M input; h input; dh_dq input; hessian input; u_des input; psi output; psi_mod output; lg_h output; H_dot output; damp input; hessian_term output; cbf output; cbf_dot output; alpha input; gamma input

function [cbf_control, psi, psi_mod,lg_h, H_dot, hessian_term, cbf, cbf_dot]= CBF(C, y, M, h, dh_dq, hessian, u_des, damp, alpha, gamma)
% Define numerical values for the parameters
    xc = 2.5;
    yc = 2;
    r = 1;

    
    m1 = 1;
    m2 = 1;
    m3 = 1;
    
    l1 = 1;
    l2 = 1;
    l3 = 1;
    
    q = reshape(y(1:3),[3,1]);
    dq = reshape(y(4:6),[3,1]);
    dh_dq = reshape(dh_dq,[1,3]);

    LIU = 1;

    if LIU == 1

    
        cbf = alpha * h + dh_dq * dq;
        lg_h = zeros(1,3);
        cbf_dot_prior = alpha .* dh_dq * dq + dq' * hessian * dq + dh_dq * (inv(M)* (-C * dq + u_des));
        psi = cbf_dot_prior + gamma .* cbf;
        if psi<0
            lg_h = dh_dq * inv(M);
            cbf_control =  - lg_h' /(lg_h * lg_h')  .* psi;
            
        else
            cbf_control = zeros(3,1);
        end
        cbf_dot = alpha .* dh_dq * dq + dq' * hessian * dq + dh_dq * inv(M)* (-C * dq + u_des+ cbf_control);
        psi_mod = cbf_dot + gamma .* cbf;

        H_dot = dq' * cbf_control - dq' * damp * dq;

        hessian_term = dq' * hessian * dq;
    
    else
        KE = 0.5 * dq' * M * dq;
        cbf = alpha * h - KE;
        lg_h = zeros(1,3);
        cbf_dot_prior = alpha .* dh_dq * dq - dq' * inv(M) * u_des;
        psi = cbf_dot_prior + gamma .* cbf;
        if psi<0
            lg_h = -dq';
            cbf_control =  dq /(dq'*dq)  .* psi;
        else
            cbf_control = zeros(3,1);
        end
        cbf_dot =  alpha .* dh_dq * dq - dq' * inv(M) * (u_des+cbf_control) ;
        psi_mod = cbf_dot + gamma .* cbf;

        H_dot = dq' * cbf_control - dq' * damp * dq;


        hessian_term = 0;
        
    end
    
end

== matlab function FInal_Liu_simulation/Subsystem/MATLAB Function18 ==
  data: y input; h output; dh_dq output; hessian_sym output
function [h, dh_dq, hessian_sym] = obstacle(y)
    % Define numerical values for the parameters
    xc = 2.5;
    yc = 2;
    r = 1;

    l1 = 1;
    l2 = 1;
    l3 = 1;
    
    % Compute the end-effector position using forward kinematics
    q1 = y(1);
    q2 = y(2);
    q3 = y(3);
    
    x_ee = l1 * cos(q1) + l2 * cos(q1 + q2) + l3 * cos(q1 + q2 + q3);
    y_ee = l1 * sin(q1) + l2 * sin(q1 + q2) + l3 * sin(q1 + q2 + q3);
    
    % Compute the control barrier function h
    h = (xc - x_ee)^2 + (yc - y_ee)^2 - r^2;
    
    % Define the expressions for dh_dq and hessian_sym
    dh_dq = [2*(cos(q1 + q2 + q3) + cos(q1 + q2) + cos(q1))*(sin(q1 + q2 + q3) + sin(q1 + q2) + sin(q1) - 2) - 2*(sin(q1 + q2 + q3) + sin(q1 + q2) + sin(q1))*(cos(q1 + q2 + q3) + cos(q1 + q2) + cos(q1) - 5/2), 2*(cos(q1 + q2 + q3) + cos(q1 + q2))*(sin(q1 + q2 + q3) + sin(q1 + q2) + sin(q1) - 2) - 2*(sin(q1 + q2 + q3) + sin(q1 + q2))*(cos(q1 + q2 + q3) + cos(q1 + q2) + cos(q1) - 5/2), 2*cos(q1 + q2 + q3)*(sin(q1 + q2 + q3) + sin(q1 + q2) + sin(q1) - 2) - 2*sin(q1 + q2 + q3)*(cos(q1 + q2 + q3) + cos(q1 + q2) + cos(q1) - 5/2)];


    hessian_sym = [                                              2*(cos(q1 + q2 + q3) + cos(q1 + q2) + cos(q1))^2 - 2*(cos(q1 + q2 + q3) + cos(q1 + q2) + cos(q1))*(cos(q1 + q2 + q3) + cos(q1 + q2) + cos(q1) - 5/2) + 2*(sin(q1 + q2 + q3) + sin(q1 + q2) + sin(q1))^2 - 2*(sin(q1 + q2 + q3) + sin(q1 + q2) + sin(q1))*(sin(q1 + q2 + q3) + sin(q1 + q2) + sin(q1) - 2), 2*(cos(q1 + q2 + q3) + cos(q1 + q2))*(cos(q1 + q2 + q3) + cos(q1 + q2) + cos(q1)) - 2*(cos(q1 + q2 + q3) + cos(q1 + q2))*(cos(q1 + q2 + q3) + cos(q1 + q2) + cos(q1) - 5/2) + 2*(sin(q1 + q2 + q3) + sin(q1 + q2))*(sin(q1 + q2 + q3) + sin(q1 + q2) + sin(q1)) - 2*(sin(q1 + q2 + q3) + sin(q1 + q2))*(sin(q1 + q2 + q3) + sin(q1 + q2) + sin(q1) - 2), 2*cos(q1 + q2 + q3)*(cos(q1 + q2 + q3) + cos(q1 + q2) + cos(q1)) - 2*cos(q1 + q2 + q3)*(cos(q1 + q2 + q3) + cos(q1 + q2) + cos(q1) - 5/2) + 2*sin(q1 + q2 + q3)*(sin(q1 + q2 + q3) + sin(q1 + q2) + sin(q1)) - 2*sin(q1 + q2 + q3)*(sin(q1 + q2 + q3) + sin(q1 + q2) + sin(q1) - 2);
        2*(cos(q1 + q2 + q3) + cos(q1 + q2))*(cos(q1 + q2 + q3) + cos(q1 + q2) + cos(q1)) - 2*(cos(q1 + q2 + q3) + cos(q1 + q2))*(cos(q1 + q2 + q3) + cos(q1 + q2) + cos(q1) - 5/2) + 2*(sin(q1 + q2 + q3) + sin(q1 + q2))*(sin(q1 + q2 + q3) + sin(q1 + q2) + sin(q1)) - 2*(sin(q1 + q2 + q3) + sin(q1 + q2))*(sin(q1 + q2 + q3) + sin(q1 + q2) + sin(q1) - 2),                                                                                       2*(cos(q1 + q2 + q3) + cos(q1 + q2))^2 - 2*(cos(q1 + q2 + q3) + cos(q1 + q2))*(cos(q1 + q2 + q3) + cos(q1 + q2) + cos(q1) - 5/2) + 2*(sin(q1 + q2 + q3) + sin(q1 + q2))^2 - 2*(sin(q1 + q2 + q3) + sin(q1 + q2))*(sin(q1 + q2 + q3) + sin(q1 + q2) + sin(q1) - 2),                     2*cos(q1 + q2 + q3)*(cos(q1 + q2 + q3) + cos(q1 + q2)) - 2*cos(q1 + q2 + q3)*(cos(q1 + q2 + q3) + cos(q1 + q2) + cos(q1) - 5/2) - 2*sin(q1 + q2 + q3)*(sin(q1 + q2 + q3) + sin(q1 + q2) + sin(q1) - 2) + 2*sin(q1 + q2 + q3)*(sin(q1 + q2 + q3) + sin(q1 + q2));
                                                                            2*cos(q1 + q2 + q3)*(cos(q1 + q2 + q3) + cos(q1 + q2) + cos(q1)) - 2*cos(q1 + q2 + q3)*(cos(q1 + q2 + q3) + cos(q1 + q2) + cos(q1) - 5/2) + 2*sin(q1 + q2 + q3)*(sin(q1 + q2 + q3) + sin(q1 + q2) + sin(q1)) - 2*sin(q1 + q2 + q3)*(sin(q1 + q2 + q3) + sin(q1 + q2) + sin(q1) - 2),                                                                                         2*cos(q1 + q2 + q3)*(cos(q1 + q2 + q3) + cos(q1 + q2)) - 2*cos(q1 + q2 + q3)*(cos(q1 + q2 + q3) + cos(q1 + q2) + cos(q1) - 5/2) - 2*sin(q1 + q2 + q3)*(sin(q1 + q2 + q3) + sin(q1 + q2) + sin(q1) - 2) + 2*sin(q1 + q2 + q3)*(sin(q1 + q2 + q3) + sin(q1 + q2)),                                                                                       2*cos(q1 + q2 + q3)^2 - 2*cos(q1 + q2 + q3)*(cos(q1 + q2 + q3) + cos(q1 + q2) + cos(q1) - 5/2) + 2*sin(q1 + q2 + q3)^2 - 2*sin(q1 + q2 + q3)*(sin(q1 + q2 + q3) + sin(q1 + q2) + sin(q1) - 2)];
     

    % d = eig(hessian_sym)
    % isposdef = all(d >= 0);
    % 
    % assert(isposdef, 'error hessian');
end

== matlab function FInal_Liu_simulation/Subsystem/MATLAB Function19 ==
  data: q_d output; y input; spring input; out output; damp input
function [q_d, out] = u_des(y, spring, damp)


    q = reshape(y(1:3),[3,1]);
    dq = reshape(y(4:6),[3,1]);

    q_d = [pi; 0; pi/4];
    
    out =  - damp * dq - spring * (q-q_d);

== matlab function FInal_Liu_simulation/Subsystem/MATLAB Function20 ==
  data: M input; E output; y input; spring input; q_d input
function E = energy(M,y,spring, q_d)
    q = y(1:3);
    dq = y(4:6);
    

    E = 0.5 * (dq' * M * dq) + 0.5 * spring *(q-q_d)' * (q-q_d);

== matlab function FInal_Liu_simulation/Subsystem/MATLAB Function21 ==
  data: M_dot input; out_1 output; S input; q input; out_2 output


function [out_1, out_2] = M_dot_coriolis_check(M_dot,S, q)
    dq = reshape(q(4:6),[3,1]);
    
    q1 = q(1);
    q2 = q(2);
    q3 = q(3);
    dq1 = q(4);
    dq2 = q(5);
    dq3 = q(6);

    check = M_dot - 2 * S;


    out_1 = dq' * check * dq;


    M_dot_formula =   [        - dq2*(sin(q2 + q3) + 3*sin(q2)) - dq3*(sin(q2 + q3) + sin(q3)), - dq3*(sin(q2 + q3)/2 + sin(q3)) - dq2*(sin(q2 + q3)/2 + (3*sin(q2))/2), - (dq2*sin(q2 + q3))/2 - dq3*(sin(q2 + q3)/2 + sin(q3)/2);
- dq3*(sin(q2 + q3)/2 + sin(q3)) - dq2*(sin(q2 + q3)/2 + (3*sin(q2))/2),                                                            -dq3*sin(q3),                                          -(dq3*sin(q3))/2;
              - (dq2*sin(q2 + q3))/2 - dq3*(sin(q2 + q3)/2 + sin(q3)/2),                                                        -(dq3*sin(q3))/2,                                                         0];
 

    
    out_2 = dq' * (M_dot_formula - 2 * S) * dq;
end

== matlab function FInal_Liu_simulation/Liu/MATLAB Function1 ==
  data: y input; M output
function M = inertia_M(y)

    q1 = y(1);
    q2 = y(2);
    q3 = y(3);

    M  = [        cos(q2 + q3) + 3*cos(q2) + cos(q3) + 4, cos(q2 + q3)/2 + (3*cos(q2))/2 + cos(q3) + 5/3, cos(q2 + q3)/2 + cos(q3)/2 + 1/3;
cos(q2 + q3)/2 + (3*cos(q2))/2 + cos(q3) + 5/3,                                  cos(q3) + 5/3,                  cos(q3)/2 + 1/3;
              cos(q2 + q3)/2 + cos(q3)/2 + 1/3,                                cos(q3)/2 + 1/3,                              1/3];

    assert(isequal(M, M'),'error')

== matlab function FInal_Liu_simulation/Subsystem/MATLAB Function22 ==
  data: u_des input; damp input; M input; y input; y output; C input; H_dot output; u_sc input; safety input; norm_u_tot output
function [y,H_dot,norm_u_tot]= dynamics(u_des, damp , M,y, C, u_sc, safety)
    
    q = reshape(y(1:3),[3,1]);
    dq = reshape(y(4:6),[3,1]);



    [~, p] = chol(M);
    decision = (p == 0);

    assert(decision, 'Inertia matrix is not positive definite');
    
    u_tot = u_des + safety * u_sc;
    norm_u_tot=norm(u_tot);
    ddq = inv(M) * (u_tot - C * dq ); % + u_sc

    H_dot = - dq' * damp * dq;

    y = [dq; ddq];

== matlab function FInal_Liu_simulation/Subsystem/MATLAB Function23 ==
  data: y input; M output
function M = inertia_M(y)

    q1 = y(1);
    q2 = y(2);
    q3 = y(3);

    M  = [        cos(q2 + q3) + 3*cos(q2) + cos(q3) + 4, cos(q2 + q3)/2 + (3*cos(q2))/2 + cos(q3) + 5/3, cos(q2 + q3)/2 + cos(q3)/2 + 1/3;
cos(q2 + q3)/2 + (3*cos(q2))/2 + cos(q3) + 5/3,                                  cos(q3) + 5/3,                  cos(q3)/2 + 1/3;
              cos(q2 + q3)/2 + cos(q3)/2 + 1/3,                                cos(q3)/2 + 1/3,                              1/3];

== matlab function FInal_Liu_simulation/Subsystem3/MATLAB Function16 ==
  data: y input; C output
function C = coriolis(y)

    q1 = y(1);
    q2 = y(2);
    q3 = y(3);
    dq1 = y(4);
    dq2 = y(5);
    dq3 = y(6);


    C = [- dq2*(sin(q2 + q3)/2 + (3*sin(q2))/2) - dq3*(sin(q2 + q3)/2 + sin(q3)/2), - dq1*(sin(q2 + q3)/2 + (3*sin(q2))/2) - dq2*(sin(q2 + q3)/2 + (3*sin(q2))/2) - dq3*(sin(q2 + q3)/2 + sin(q3)/2), - dq1*(sin(q2 + q3)/2 + sin(q3)/2) - dq2*(sin(q2 + q3)/2 + sin(q3)/2) - dq3*(sin(q2 + q3)/2 + sin(q3)/2);
                dq1*(sin(q2 + q3)/2 + (3*sin(q2))/2) - (dq3*sin(q3))/2,                                                                                                 -(dq3*sin(q3))/2,                                                    - (dq1*sin(q3))/2 - (dq2*sin(q3))/2 - (dq3*sin(q3))/2;
                       dq1*(sin(q2 + q3)/2 + sin(q3)/2) + (dq2*sin(q3))/2,                                                                                (dq1*sin(q3))/2 + (dq2*sin(q3))/2,                                                                                                        0];

== matlab function FInal_Liu_simulation/Subsystem3/MATLAB Function17 ==
  data: C input; y input; cbf_control output; M input; h input; dh_dq input; hessian input; u_des input; psi output; psi_mod output; lg_h output; H_dot output; damp input; hessian_term output; cbf output; cbf_dot output; alpha input; gamma input

function [cbf_control, psi, psi_mod,lg_h, H_dot, hessian_term, cbf, cbf_dot]= CBF(C, y, M, h, dh_dq, hessian, u_des, damp, alpha, gamma)
% Define numerical values for the parameters
    xc = 2.5;
    yc = 2;
    r = 1;


    
    m1 = 1;
    m2 = 1;
    m3 = 1;
    
    l1 = 1;
    l2 = 1;
    l3 = 1;
    
    q = reshape(y(1:3),[3,1]);
    dq = reshape(y(4:6),[3,1]);
    dh_dq = reshape(dh_dq,[1,3]);

    LIU = 1;

    if LIU == 1

    
        cbf = alpha * h + dh_dq * dq;
        lg_h = zeros(1,3);
        cbf_dot_prior = alpha .* dh_dq * dq + dq' * hessian * dq + dh_dq * (inv(M)* (-C * dq + u_des));
        psi = cbf_dot_prior + gamma .* cbf;
        if psi<0
            lg_h = dh_dq * inv(M);
            cbf_control =  - lg_h' /(lg_h * lg_h')  .* psi;
            
        else
            cbf_control = zeros(3,1);
        end
        cbf_dot = alpha .* dh_dq * dq + dq' * hessian * dq + dh_dq * inv(M)* (-C * dq + u_des+ cbf_control);
        psi_mod = cbf_dot + gamma .* cbf;

        H_dot = dq' * cbf_control - dq' * damp * dq;

        hessian_term = dq' * hessian * dq;
    
    else
        KE = 0.5 * dq' * M * dq;
        cbf = alpha * h - KE;
        lg_h = zeros(1,3);
        cbf_dot_prior = alpha .* dh_dq * dq - dq' * inv(M) * u_des;
        psi = cbf_dot_prior + gamma .* cbf;
        if psi<0
            lg_h = -dq';
            cbf_control =  dq /(dq'*dq)  .* psi;
        else
            cbf_control = zeros(3,1);
        end
        cbf_dot =  alpha .* dh_dq * dq - dq' * inv(M) * (u_des+cbf_control) ;
        psi_mod = cbf_dot + gamma .* cbf;

        H_dot = dq' * cbf_control - dq' * damp * dq;


        hessian_term = 0;
        
    end
    
end
